simulink model "PVArray(wrong)"  (R2016a)
settings: Solver=ode5  StartTime=0.0  StopTime=0.1  FixedStep=2e-6  MaxStep=5e-6  RelTol=1e-3
values from neighbouring files (symbols this model uses):
  C1 = t_PWM * Impp*0.1/ (8 * Vmpp*0.001)    [SolarPanelModel.m]
  C2 = Vo * t_PWM/ (Load * Vo*0.01)    [SolarPanelModel.m]
  delta_Il = Impp*0.1/ 2    [SolarPanelModel.m]
  Io = (Isc - (Voc - Rs*Isc)/ Rsh) * exp(-Voc/ (m*Vt))    [SolarPanelModel.m]
  Is = Io * exp(Voc/ (m*Vt)) + Voc/ Rsh    [SolarPanelModel.m]
  Isc = G/ Gr * (Iscr + miu_Isc*(Tc - Tr))    (= 9.386)    [SolarPanelModel.m]
  k_v = 1/ (t_PWM*100)    (= 500)    [SolarPanelModel.m]
  k_vc = 1/ (t_PWM*10)    (= 5000)    [SolarPanelModel.m]
  L_inductor = Vo * t_PWM/ (4 * Impp*0.1)    [SolarPanelModel.m]
  Load = Vo^2/Pmpp    [SolarPanelModel.m]
  m = sol(1)    [SolarPanelModel.m]
  Rs = sol(3)    [SolarPanelModel.m]
  Rsh = sol(2)    [SolarPanelModel.m]
  t_PWM = 20e-6    (= 2e-05)    [SolarPanelModel.m]
  Voc = Vocr + miu_Voc*(Tc - Tr) + m*Vt*log(G/Gr)    [SolarPanelModel.m]
  Vt = K*Tc/ q    (= 0.0291654375)    [SolarPanelModel.m]
libraries: powerlib x17, powerlib_meascontrol x2
settings Model: Creator=frede  LastModifiedBy=frede
settings DataIOCC: LimitDataPoints=on  SaveFormat=Array
settings HardwareCC: ProdBitPerPointer=32  ProdLargestAtomicFloat=None  ProdIntDivRoundTo=Undefined  ProdEndianess=Unspecified  ProdWordSize=32  ProdHWDeviceType=32-bit Generic
settings ModelReferenceCC: PropagateSignalLabelsOutOfModel=off
settings ConfigComp: CovModelRefEnable=Off

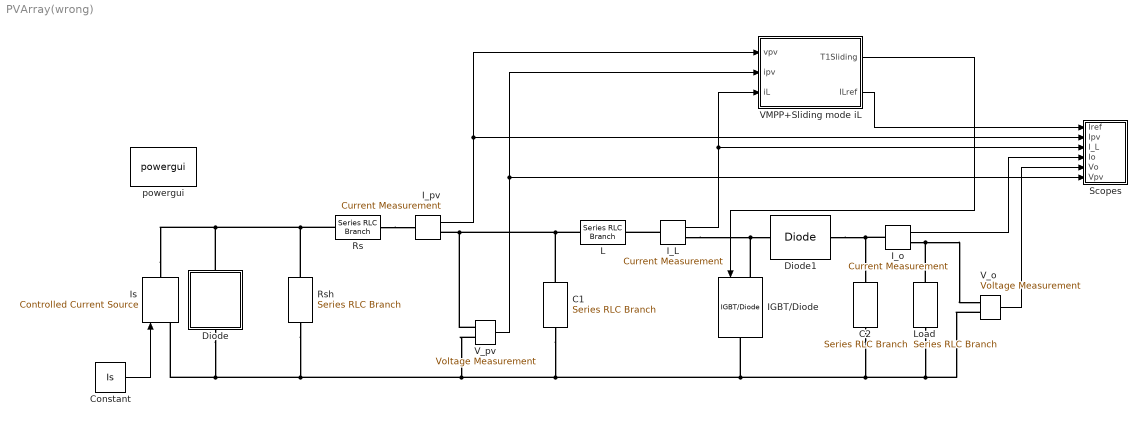
== system PVArray(wrong) ==
  C1 : powerlib/Elements/Series RLC Branch  LConnTagsString=__new0  RConnTagsString=__new0  BranchType=C  Resistance=Rs  Inductance=1e-3  SetiL0=off  InitialCurrent=0  Capacitance=C1  Setx0=off  InitialVoltage=0  Measurements=None
  C2 : powerlib/Elements/Series RLC Branch  LConnTagsString=__new0  RConnTagsString=__new0  BranchType=C  Resistance=Rs  Inductance=1e-3  SetiL0=off  InitialCurrent=0  Capacitance=C2  Setx0=off  InitialVoltage=0  Measurements=None
  Constant : Constant  Value=Is
  Diode : Subsystem  AncestorBlock=re_lib/Solar/PV Array/Diode Rsh
      mask Display:
      | plot(-75,-50,100,150, [-15 -15 43 -15 -15 -75],[50 8 50 92 50 50], ...
      |     [43 43],[8 94],[100 43], [50 50])
  Diode1 : powerlib/Power Electronics/Diode  Ron=0.001  Lon=0  Vf=0.6  IC=0  UseSnubber=off  Rs=600  Cs=2e-8  Measurements=off
  IGBT/Diode : powerlib/Power Electronics/IGBT//Diode  Ron=0.001  Rs=600  Cs=2e-8  Measurements=off
  I_L : powerlib/Measurements/Current Measurement  PhasorSimulation=off  OutputType=Complex  PSBequivalent=0
  I_o : powerlib/Measurements/Current Measurement  PhasorSimulation=off  OutputType=Complex  PSBequivalent=0
  I_pv : powerlib/Measurements/Current Measurement  PhasorSimulation=off  OutputType=Complex  PSBequivalent=0
  Is : powerlib/Electrical Sources/Controlled Current Source  Initialize=on  Source_Type=DC  Amplitude=0  Phase=0  Frequency=0  Measurements=None
  L : powerlib/Elements/Series RLC Branch  LConnTagsString=__new0  RConnTagsString=__new0  BranchType=L  Resistance=Rs  Inductance=L_inductor  SetiL0=off  InitialCurrent=0  Capacitance=1e-6  Setx0=off  InitialVoltage=0  Measurements=None
  Load : powerlib/Elements/Series RLC Branch  LConnTagsString=__new0  RConnTagsString=__new0  BranchType=R  Resistance=Load  Inductance=1e-3  SetiL0=off  InitialCurrent=0  Capacitance=1e-6  Setx0=off  InitialVoltage=0  Measurements=None
  Rs : powerlib/Elements/Series RLC Branch  LConnTagsString=__new0  RConnTagsString=__new0  BranchType=R  Resistance=Rs  Inductance=1e-3  SetiL0=off  InitialCurrent=0  Capacitance=1e-6  Setx0=off  InitialVoltage=0  Measurements=None
  Rsh : powerlib/Elements/Series RLC Branch  LConnTagsString=__new0  RConnTagsString=__new0  BranchType=R  Resistance=Rsh  Inductance=1e-3  SetiL0=off  InitialCurrent=0  Capacitance=1e-6  Setx0=off  InitialVoltage=0  Measurements=None
  Scopes : Subsystem
  VMPP+Sliding mode iL : Subsystem
  V_o : powerlib/Measurements/Voltage Measurement  PhasorSimulation=off  OutputType=Complex  PSBequivalent=0
  V_pv : powerlib/Measurements/Voltage Measurement  PhasorSimulation=off  OutputType=Complex  PSBequivalent=0
  powergui : powerlib/powergui  Priority=1  SimulationMode=Discrete  SolverType=Tustin/Backward Euler (TBE)  SampleTime=2e-6  frequency=60  SPID=off  DisableSnubberDevices=off  DisableRonSwitches=off  DisableVfSwitches=off  SwTol=0  DisplayEquations=off  Interpol=off  ExternalGateDelay=off  methode=off  Ts=10  FunctionMessages=off  echomessages=off  HookPort=off  EnableUseOfTLC=off  x0status=blocks  frequencyindice=0  Pbase=100e6  ErrMax=1e-4  Iterations=50  UnitsV=kV  UnitsW=MW  buscounter=0  RestoreLinks=warning  ResistiveCurrentMeasurement=off  Frange=[0:2:500]  Ylog=off  Xlog=on  ShowGrid=off  save=off  variable=ZData  structure=0  ZoomFFT=off  StartTime=0.0  cycles=1  DisplayStyle=1  fundamental=60  FreqAxis=off  MaxFrequency=1000  frequencyindicesteady=1  RmsSteady=1  display=off
  wires:
  VMPP+Sliding mode iL/2(ILref) -> Scopes/1(Iref)
  Constant/1 -> Is/1
  I_L/1 -> VMPP+Sliding mode iL/3(iL), Scopes/3(I_L)
  I_pv/1 -> VMPP+Sliding mode iL/1(vpv), Scopes/2(Ipv)
  I_o/1 -> Scopes/4(Io)
  V_o/1 -> Scopes/5(Vo)
  VMPP+Sliding mode iL/1(T1Sliding) -> IGBT/Diode/1
  V_pv/1 -> VMPP+Sliding mode iL/2(ipv), Scopes/6(Vpv)
  connections:
  Is/LConn1 -- Diode/RConn1 -- Rsh/RConn1 -- C2/RConn1 -- Load/RConn1 -- V_o/LConn2 -- IGBT/Diode/RConn1 -- C1/RConn1 -- V_pv/LConn2
  Is/RConn1 -- Diode/LConn1 -- Rs/LConn1 -- Rsh/LConn1
  I_pv/RConn1 -- V_pv/LConn1 -- C1/LConn1 -- L/LConn1
  I_L/RConn1 -- IGBT/Diode/LConn1 -- Diode1/LConn1
  C2/LConn1 -- Diode1/RConn1 -- I_o/LConn1
  I_o/RConn1 -- Load/LConn1 -- V_o/LConn1
  I_L/LConn1 -- L/RConn1
  Rs/RConn1 -- I_pv/LConn1

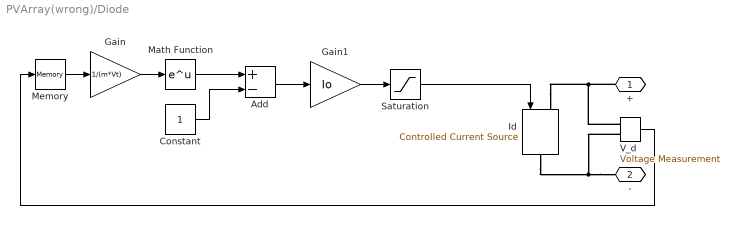
== system PVArray(wrong)/Diode ==
  Add : Sum  Inputs=+-
  Constant : Constant
  Gain : Gain  Gain=1/(m*Vt)
  Gain1 : Gain  Gain=Io
  Id : powerlib/Electrical Sources/Controlled Current Source  Initialize=on  Source_Type=DC  Amplitude=200  Phase=0  Frequency=0  Measurements=None
  Math Function : Math  SaturateOnIntegerOverflow=on
  Memory : Memory
  Saturation : Saturate  UpperLimit=Isc  LowerLimit=0
  V_d : powerlib/Measurements/Voltage Measurement  PhasorSimulation=off  OutputType=Complex  PSBequivalent=0
  + : PMIOPort  Port=1  Side=Left
  - : PMIOPort  Port=2  Side=Right
  wires:
  Math Function/1 -> Add/1
  Gain/1 -> Math Function/1
  Constant/1 -> Add/2
  Add/1 -> Gain1/1
  V_d/1 -> Memory/1
  Memory/1 -> Gain/1
  Saturation/1 -> Id/1
  Gain1/1 -> Saturation/1
  connections:
  -/RConn1 -- Id/RConn1 -- V_d/LConn2
  Id/LConn1 -- +/RConn1 -- V_d/LConn1

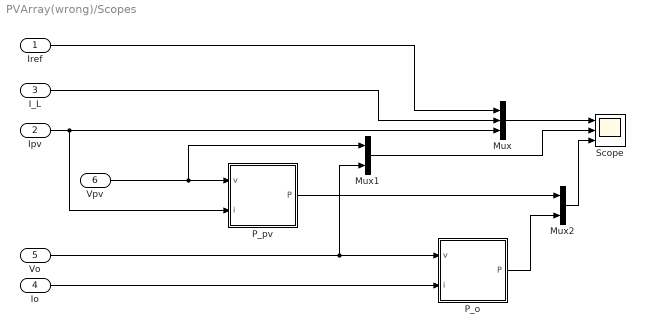
== system PVArray(wrong)/Scopes ==
  Iref : Inport
  Ipv : Inport  Port=2
  I_L : Inport  Port=3
  Io : Inport  Port=4
  Vo : Inport  Port=5
  Vpv : Inport  Port=6
  Mux : Mux  Inputs=3
  Mux1 : Mux  Inputs=2
  Mux2 : Mux  Inputs=2
  P_o : Subsystem
  P_pv : Subsystem
  Scope : Scope  NumInputPorts=3
  wires:
  Mux/1 -> Scope/1
  P_o/1(P) -> Mux2/2
  Mux2/1 -> Scope/3
  P_pv/1(P) -> Mux2/1
  Io/1 -> P_o/2(i)
  Mux1/1 -> Scope/2
  I_L/1 -> Mux/2
  Vo/1 -> P_o/1(v), Mux1/2
  Ipv/1 -> Mux/3, P_pv/2(i)
  Vpv/1 -> P_pv/1(v), Mux1/1
  Iref/1 -> Mux/1

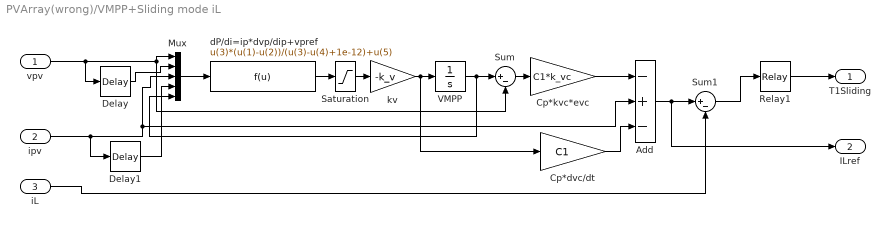
== system PVArray(wrong)/VMPP+Sliding mode iL ==
  vpv : Inport
  ipv : Inport  Port=2
  iL : Inport  Port=3
  Add : Sum  Inputs=-+-
  Cp*dvc/dt : Gain  Gain=C1
  Cp*kvc*evc : Gain  Gain=C1*k_vc
  Delay : TransportDelay  DelayTime=t_PWM/10
  Delay1 : TransportDelay  DelayTime=t_PWM/10
  Mux : Mux  Inputs=5
  Relay1 : Relay  OnSwitchValue=delta_Il  OffSwitchValue=-delta_Il  ZeroCross=off
  Saturation : Saturate  UpperLimit=1  LowerLimit=-1  ZeroCross=off
  Sum : Sum  Inputs=|+-
  Sum1 : Sum  Inputs=|+-
  VMPP : Integrator  InitialCondition=Voc*0.75  LimitOutput=on  UpperSaturationLimit=Voc  LowerSaturationLimit=Voc/4
  dP/di=ip*dvp/dip+vpref : Fcn  Expr=u(3)*(u(1)-u(2))/(u(3)-u(4)+1e-12)+u(5)
  kv : Gain  Gain=-k_v
  T1Sliding : Outport
  ILref : Outport  Port=2
  wires:
  kv/1 -> Cp*dvc/dt/1, VMPP/1
  Saturation/1 -> kv/1
  VMPP/1 -> Mux/5, Sum/1
  vpv/1 -> Sum/2, Mux/1, Delay/1
  Delay/1 -> Mux/2
  Delay1/1 -> Mux/4
  Mux/1 -> dP/di=ip*dvp/dip+vpref/1
  dP/di=ip*dvp/dip+vpref/1 -> Saturation/1
  Relay1/1 -> T1Sliding/1
  ipv/1 -> Delay1/1, Add/2, Mux/3
  Sum/1 -> Cp*kvc*evc/1
  Add/1 -> ILref/1, Sum1/1
  iL/1 -> Sum1/2
  Sum1/1 -> Relay1/1
  Cp*kvc*evc/1 -> Add/1
  Cp*dvc/dt/1 -> Add/3

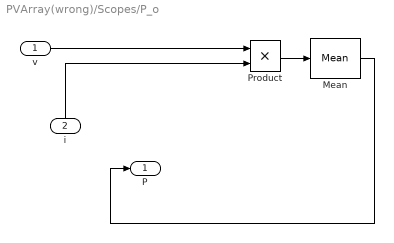
== system PVArray(wrong)/Scopes/P_o ==
  v : Inport
  i : Inport  Port=2
  Mean : powerlib_meascontrol/Measurements/Mean  Freq=100  Vinit=230  Ts=0
  Product : Product
  P : Outport
  wires:
  i/1 -> Product/2
  v/1 -> Product/1
  Product/1 -> Mean/1
  Mean/1 -> P/1

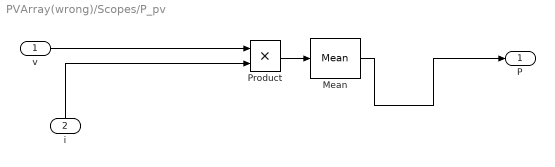
== system PVArray(wrong)/Scopes/P_pv ==
  v : Inport
  i : Inport  Port=2
  Mean : powerlib_meascontrol/Measurements/Mean  Freq=100  Vinit=230  Ts=0
  Product : Product
  P : Outport
  wires:
  Mean/1 -> P/1
  Product/1 -> Mean/1
  v/1 -> Product/1
  i/1 -> Product/2
